simulink model "pic8"  (R2025b)
settings: Solver=ode45  StartTime=0.0  StopTime=10.0  MaxStep=0.01  RelTol=1e-3
undefined symbols (not defined in the file or in its folder): K_FB
settings Model: Creator=Nickolay  LastModifiedBy=Nickolay

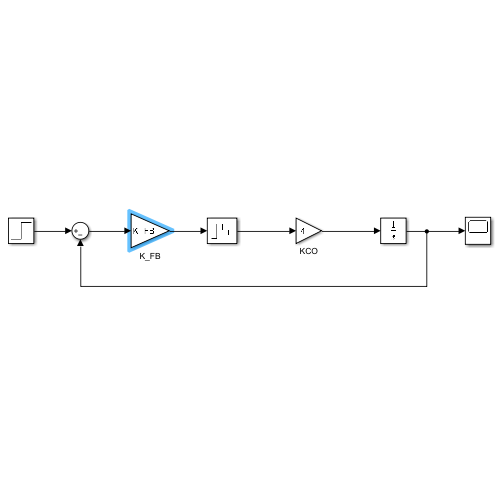
[thumbnail: Simulink's stored preview of the top-level diagram]
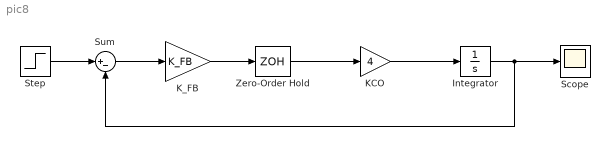
== system pic8 ==
  Integrator : Integrator
  KCO : Gain  Gain=4
  K_FB : Gain  Gain=K_FB
  Scope : Scope
  Step : Step  Time=0  SampleTime=0
  Sum : Sum  Inputs=|+-
  Zero-Order Hold : ZeroOrderHold  SampleTime=0.2
  wires:
  Step/1 -> Sum/1
  Sum/1 -> K_FB/1
  K_FB/1 -> Zero-Order Hold/1
  Zero-Order Hold/1 -> KCO/1
  KCO/1 -> Integrator/1
  Integrator/1 -> Sum/2, Scope/1
